simulink library "My_library"  (R2018a)
settings: Solver=VariableStepAuto  StartTime=0.0  StopTime=10.0  RelTol=1e-3  EnableMultiTasking=on
undefined symbols (not defined in the file or in its folder): Ax, Ay, Az, gn, Newton, Nx, Ny, Nz, Raphson, Rx, Ry, Rz, st
libraries: $bdroot x11, simulink x1
(part 1 of 2)
settings Model: Creator=Navya  LastModifiedBy=IGOSAT
settings DataIOCC: LimitDataPoints=on
settings OptimizationCC: LifeSpan=inf
settings DebuggingCC: AllowSymbolicDim=off  SFUnexpectedBacktrackingDiag=warning  SFNoUnconditionalDefaultTransitionDiag=warning  SFExecutionAtInitializationDiag=none
settings ModelReferenceCC: PropagateSignalLabelsOutOfModel=off
settings CodeAppCC: StateflowObjectComments=on
settings GRTTargetCC: TargetLangStandard=C89/C90 (ANSI)
settings ConfigComp: CovMetricSettings=dw  CovHtmlReporting=on  CovSaveCumulativeToWorkspaceVar=on  CovSaveSingleToWorkspaceVar=on  CovExternalEMLEnable=off

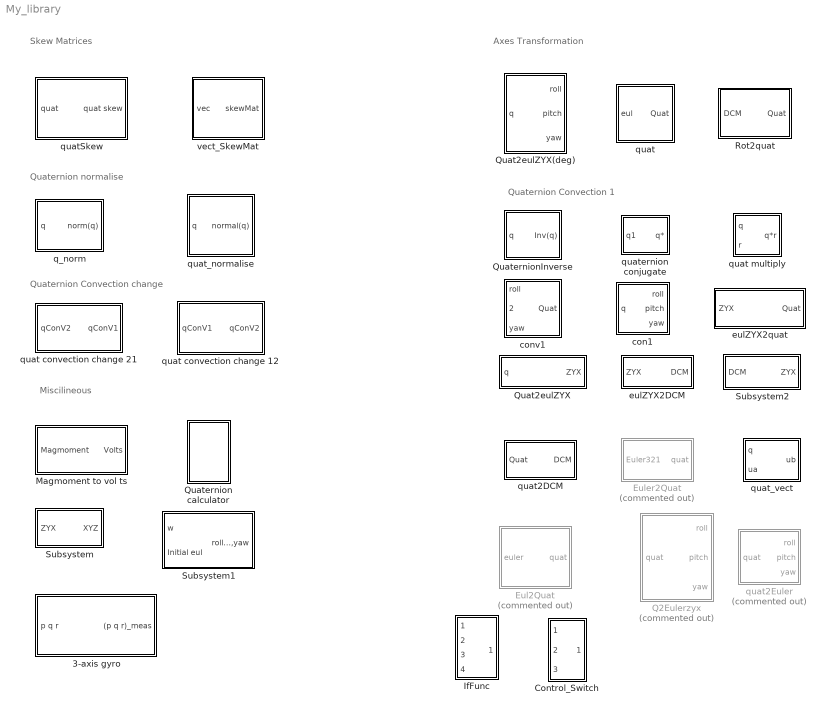
== system My_library ==
  note: Quaternion Convection 1
  note: Miscilineous
  note: Axes Transformation
  note: Quaternion Convection change
  note: Quaternion normalise
  note: Skew Matrices
  3-axis gyro : Subsystem  mask{dtype_g=off, w_g=190, z_g=0.707, g_sf_cc=[1 0 0; 0 1 0; 0 0 1], g_bias=1e-4*[1 1 1], g_sen=[0 0 0], g_Ts=0, Gs=0, g_rand=on, g_seeds=[23093 23094 23095], g_pow=gn, g_sat=[-inf  -inf  -inf  inf inf inf], ts=st}
      mask prompts: dtype_g "Second-order dynamics"; w_g "Natural frequency (rad/sec):"; z_g "Damping ratio:"; g_sf_cc "Scale factors and cross-coupling:"; g_bias "Measurement bias:"; g_sen "G-sensitive bias:"; g_Ts "Update rate (sec):"; Gs "Gyro sensitivity"; g_rand "Noise on:"; g_seeds "Noise seeds:"; g_pow "Noisepower:"; g_sat "Lower and upper output limits:"; ts "sampling time"
      mask init:
      | par = g_Ts;
      | block = gcb;
      | g_satl = g_sat(1:3);
      | g_sath = g_sat(4:6);
      | Ts=ts;
      mask DialogControl ParameterTabVar0 Prompt: Main
      mask DialogControl ParameterTabVar01 Prompt: Noise
      mask Display:
      | port_label('input',1,'w (rad/s)')
      | port_label('output',1,'w_meas (rad/s)')
  "Control_Switch " : Subsystem
  Eul2Quat : Subsystem  Commented=on
      mask help:
      | Converts euler(in deg) to Quaternion(of convection 2).
      | Input  : 3 x 1 [roll;pitch;yaw]
      | Output : 4 x 1
  Euler2Quat : Subsystem  Commented=on
      mask help: Convert euler321(in radians) to Quaternion of convection-2
  "IfFunc " : Subsystem
  Magmoment to vol ts : Subsystem
  Q2Eulerzyx : Subsystem  Commented=on
      mask help: Quaternion(convention 2) to euler(roll,pitch, yaw) in degress
  Quat2eulZYX : Subsystem
      mask help: Quaternion(Conv1) to euler ZYX(in rad)
  Quat2eulZYX(deg) : Subsystem
      mask help: Quaternion(convention 2) to euler(roll,pitch, yaw) in degress
  Quaternion calculator : Subsystem
      mask help: Calculates quaternion of convention-2 from euler angles
  QuaternionInverse : Subsystem
      mask help: Computes quaternion inverse for conv-1
  Rot2quat : Subsystem
      mask help: Rotation matrix to quaternion (conv-1)
  Subsystem : Subsystem
      mask help: Converts XYZ to ZYX format or viceversa
  Subsystem1 : Subsystem
      mask help: Computes euler angles (roll, pitch, yaw) from anguler rates(wx,wy,wz)
  Subsystem2 : Subsystem
      mask help: Converts DCM to euler ZYX
  con1 : Subsystem
      mask help: Quaternion(convention 1) to euler(roll,pitch, yaw) in degress
  conv1 : Subsystem
      mask help: roll pitch yaw(in rad) to quaternion conv-1 based on ZYX transformation
  eulZYX2DCM : Subsystem
      mask help: eulZYX(in rad) to DM
  eulZYX2quat : Subsystem
      mask help: euler ZYX(in rad) to Quaternion(Conv1).
  q_norm : Subsystem
      mask help:
      | Computes quaternion norm
      | norm(q) = q1^2+q2^2+q3^2+q4^2
  quat : Subsystem
      mask help:
      | Converts roll, pitch, yaw (in degress) to quaternion conv-2 based on eulZYX
      | Inputs: roll
      |         pitch
      |         yaw
      | Outputs:Quaternion [eps, eta]'
  quat convection change 12 : Subsystem
      mask help:
      | Changes the quaternion convection from 1 to 2
      | [q0;q1;q2;q3]->[q1;q2;q3;q4]
  quat convection change 21 : Subsystem
      mask help:
      | Changes the quaternion convection from 2 to 1
      | [q1;q2;q3;q4]->[q0;q1;q2;q3]
  quat multiply : Subsystem
      mask help:
      | quaternion multiplication (for conv-1)
      | qr = q*r
  quat2DCM : Subsystem
      mask help: Quaternion(conv - 1) to rotational matrix
  quat2Euler : Subsystem  Commented=on
      mask help: Converts quaternion(conv-2) to Euler Angles(in rad)
  quatSkew : Subsystem
      mask help: Compute quaternion skew matrix
  quat_normalise : Subsystem
      mask help:
      | Normalises the quaternion
      | normal(q)= q/√norm(q)
  quat_vect : Subsystem
      mask help:
      | If q is convention-1 and it tranforms vector from a to b.
      | ub = qba * ua
  quaternion conjugate : Subsystem
      mask help: Quaternion conjugate for convection-1
  vect_SkewMat : Subsystem
      mask help: Computes 3x3 skew matrix of a vector

== system My_library/3-axis gyro ==
  p q r : Inport  PortDimensions=3
  Measurement bias : Constant  Value=g_bias
  Product : Product  Multiplication=Matrix(*)  SaturateOnIntegerOverflow=on  OutDataTypeStr=Inherit: Same as first input
  Product1 : Product  SaturateOnIntegerOverflow=on  OutDataTypeStr=Inherit: Same as first input
  Random bias : simulink/Sources/Band-Limited White Noise  Cov=g_pow  Ts=Ts  seed=g_seeds(1:3)
  Saturation : Saturate  UpperLimit=g_sath  LowerLimit=g_satl
  "Scale factors & Cross-coupling errors " : Constant  Value=g_sf_cc
  Subsystem : Subsystem
  Sum1 : Sum  Inputs=|++  SaturateOnIntegerOverflow=on
  Sum4 : Sum  Inputs=+++  SaturateOnIntegerOverflow=on
  Zero-Order Hold : Gain  SaturateOnIntegerOverflow=on  OutDataTypeStr=Inherit: Same as input  ParamDataTypeStr=Inherit: Same as input
  Zero-Order Hold1 : Gain  SaturateOnIntegerOverflow=on  OutDataTypeStr=Inherit: Same as input  ParamDataTypeStr=Inherit: Same as input
  g-sensitive bias : Constant  Value=g_sen
  gyro sensitivity : Constant  Value=Gs
  (p q r)_meas : Outport
  wires:
  Sum4/1 -> Subsystem/1(p q r)
  "Scale factors & Cross-coupling errors "/1 -> Product/1
  p q r/1 -> Zero-Order Hold/1
  Subsystem/1("p q r ") -> Sum1/1
  Sum1/1 -> Saturation/1
  Zero-Order Hold/1 -> Product/2
  Saturation/1 -> (p q r)_meas/1
  g-sensitive bias/1 -> Product1/2
  Measurement bias/1 -> Sum4/2
  Product/1 -> Sum4/1
  Zero-Order Hold1/1 -> Product1/1
  Product1/1 -> Sum4/3
  gyro sensitivity/1 -> Zero-Order Hold1/1
  Random bias/1 -> Sum1/2

== system My_library/Control_Switch  ==
  In1 : Inport
  In2 : Inport  Port=2
  In3 : Inport  Port=3
  Control switch : Switch  Criteria=u2 ~= 0  Threshold=10000
  MATLAB Function2 : MATLAB Function  TreatAsAtomicUnit=on
  Out1 : Outport
  wires:
  In3/1 -> Control switch/3
  In1/1 -> Control switch/1
  In2/1 -> MATLAB Function2/1(x)
  Control switch/1 -> Out1/1
  MATLAB Function2/1(yes) -> Control switch/2

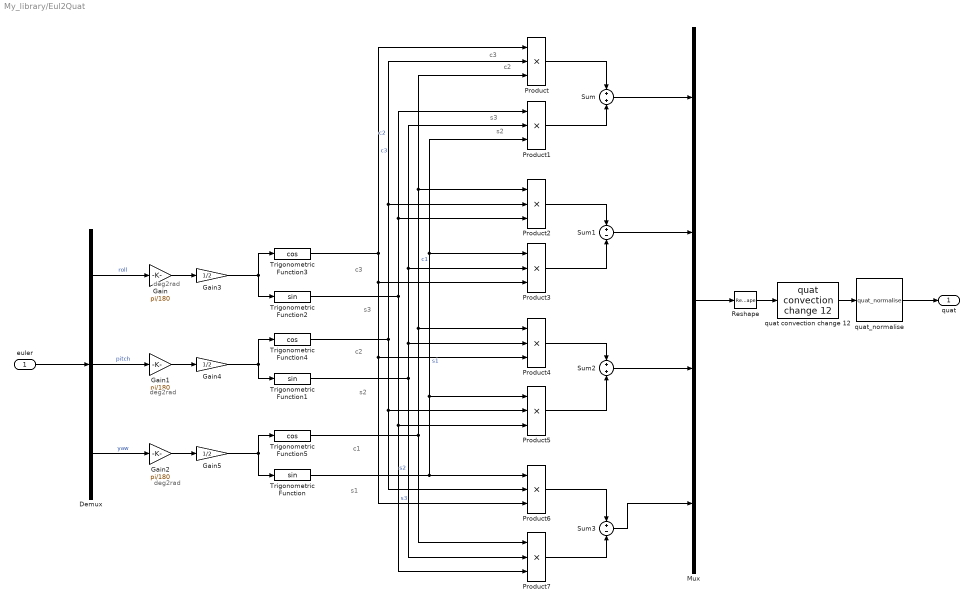
== system My_library/Eul2Quat ==
  note: deg2rad
  note: deg2rad
  note: deg2rad
  note: c2
  note: c3
  note: s2
  note: s3
  note: s1
  note: c1
  note: s2
  note: c2
  note: s3
  note: c3
  euler : Inport
  Demux : Demux  Outputs=3
  Gain : Gain  Gain=pi/180
  Gain1 : Gain  Gain=pi/180
  Gain2 : Gain  Gain=pi/180
  Gain3 : Gain  Gain=1/2
  Gain4 : Gain  Gain=1/2
  Gain5 : Gain  Gain=1/2
  Mux : Mux
  Product{,1..7} (8 alike) : Product  Inputs=3
  Reshape : Reshape
  Sum : Sum  Inputs=+|+
  Sum1 : Sum  Inputs=+|-
  Sum2 : Sum  Inputs=+|+
  Sum3 : Sum  Inputs=+|-
  Trigonometric Function : Trigonometry
  Trigonometric Function1 : Trigonometry
  Trigonometric Function2 : Trigonometry
  Trigonometric Function3 : Trigonometry  Operator=cos
  Trigonometric Function4 : Trigonometry  Operator=cos
  Trigonometric Function5 : Trigonometry  Operator=cos
  quat convection change 12 : $bdroot/quat convection change 12
  quat_normalise : $bdroot/quat_normalise
  quat : Outport
  wires:
  Gain1/1 -> Gain4/1
  Trigonometric Function2/1 -> Product2/3, Product1/1, Product7/3, Product5/3  "s3"
  Product2/1 -> Sum1/1
  Trigonometric Function3/1 -> Product/1, Product6/3, Product4/3, Product3/3  "c3"
  Sum/1 -> Mux/1
  Product3/1 -> Sum1/2
  Product1/1 -> Sum/2
  Product4/1 -> Sum2/1
  Trigonometric Function4/1 -> Product2/2, Product/2, Product6/2, Product5/2  "c2"
  Sum2/1 -> Mux/3
  Product7/1 -> Sum3/2
  Trigonometric Function1/1 -> Product4/2, Product1/2, Product3/2, Product7/2  "s2"
  Product/1 -> Sum/1
  Product6/1 -> Sum3/1
  Sum3/1 -> Mux/4
  Gain4/1 -> Trigonometric Function4/1, Trigonometric Function1/1
  Gain3/1 -> Trigonometric Function2/1, Trigonometric Function3/1
  Product5/1 -> Sum2/2
  Gain5/1 -> Trigonometric Function/1, Trigonometric Function5/1
  euler/1 -> Demux/1
  Mux/1 -> Reshape/1
  Trigonometric Function5/1 -> Product7/1, Product4/1, Product2/1, Product/3  "c1"
  Sum1/1 -> Mux/2
  Demux/1 -> Gain/1  "roll"
  Demux/3 -> Gain2/1  "yaw"
  Gain/1 -> Gain3/1
  Gain2/1 -> Gain5/1
  Trigonometric Function/1 -> Product3/1, Product1/3, Product5/1, Product6/1  "s1"
  Demux/2 -> Gain1/1  "pitch"
  Reshape/1 -> quat convection change 12/1
  quat convection change 12/1 -> quat_normalise/1
  quat_normalise/1 -> quat/1

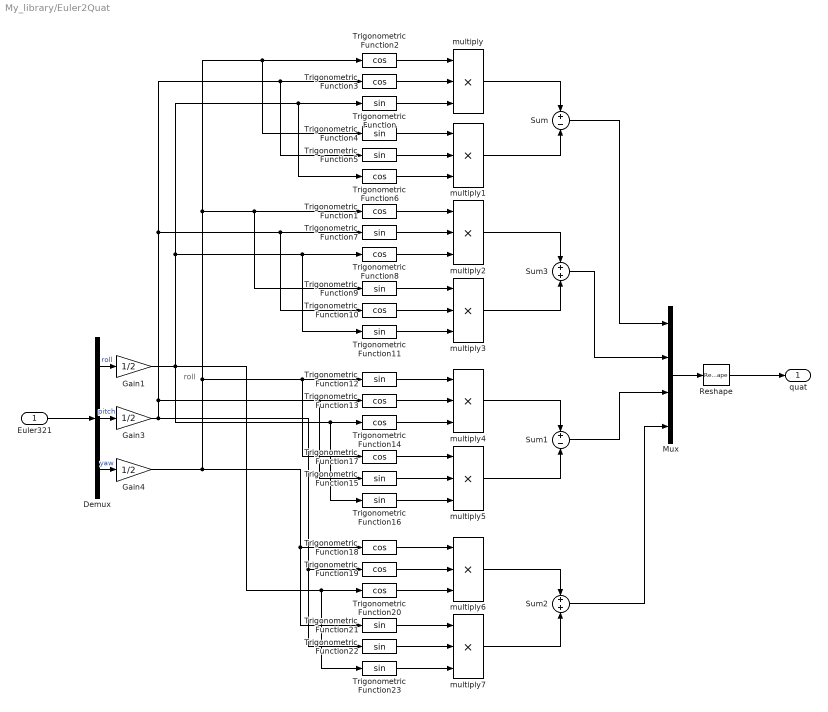
== system My_library/Euler2Quat ==
  note: roll
  Euler321 : Inport
  Demux : Demux  Outputs=3
  Gain1 : Gain  Gain=1/2
  Gain3 : Gain  Gain=1/2
  Gain4 : Gain  Gain=1/2
  Mux : Mux
  Reshape : Reshape
  Sum : Sum  Inputs=+-
  Sum1 : Sum  Inputs=+-
  Sum2 : Sum
  Sum3 : Sum
  Trigonometric Function{,4..5,7,9,11..12,15..16,21..23} (12 alike) : Trigonometry
  Trigonometric Function{1..3,6,8,10,13..14,17..20} (12 alike) : Trigonometry  Operator=cos
  multiply{,1..7} (8 alike) : Product  Inputs=***
  quat : Outport
  wires:
  Trigonometric Function1/1 -> multiply2/1
  Trigonometric Function9/1 -> multiply3/1
  Demux/2 -> Gain3/1  "pitch"
  multiply6/1 -> Sum2/1
  Euler321/1 -> Demux/1
  Trigonometric Function8/1 -> multiply2/3
  Demux/3 -> Gain4/1  "yaw"
  Trigonometric Function5/1 -> multiply1/2
  Trigonometric Function4/1 -> multiply1/1
  Trigonometric Function14/1 -> multiply4/3
  multiply1/1 -> Sum/2
  Trigonometric Function12/1 -> multiply4/1
  Trigonometric Function3/1 -> multiply/2
  Trigonometric Function13/1 -> multiply4/2
  Trigonometric Function6/1 -> multiply1/3
  Gain1/1 -> Trigonometric Function23/1, Trigonometric Function20/1, Trigonometric Function16/1, Trigonometric Function14/1, Trigonometric Function11/1, Trigonometric Function8/1, Trigonometric Function6/1, Trigonometric Function/1
  Gain3/1 -> Trigonometric Function22/1, Trigonometric Function19/1, Trigonometric Function15/1, Trigonometric Function13/1, Trigonometric Function10/1, Trigonometric Function7/1, Trigonometric Function5/1, Trigonometric Function3/1
  Gain4/1 -> Trigonometric Function21/1, Trigonometric Function18/1, Trigonometric Function17/1, Trigonometric Function12/1, Trigonometric Function4/1, Trigonometric Function2/1, Trigonometric Function9/1, Trigonometric Function1/1
  multiply7/1 -> Sum2/2
  Trigonometric Function23/1 -> multiply7/3
  Trigonometric Function2/1 -> multiply/1
  Mux/1 -> Reshape/1
  multiply3/1 -> Sum3/2
  Trigonometric Function16/1 -> multiply5/3
  Sum1/1 -> Mux/3
  Trigonometric Function22/1 -> multiply7/2
  multiply5/1 -> Sum1/2
  multiply/1 -> Sum/1
  Trigonometric Function15/1 -> multiply5/2
  Trigonometric Function17/1 -> multiply5/1
  Sum2/1 -> Mux/4
  Trigonometric Function10/1 -> multiply3/2
  Trigonometric Function21/1 -> multiply7/1
  Trigonometric Function/1 -> multiply/3
  multiply4/1 -> Sum1/1
  Reshape/1 -> quat/1
  Trigonometric Function18/1 -> multiply6/1
  Trigonometric Function20/1 -> multiply6/3
  Sum/1 -> Mux/1
  Trigonometric Function19/1 -> multiply6/2
  multiply2/1 -> Sum3/1
  Sum3/1 -> Mux/2
  Trigonometric Function7/1 -> multiply2/2
  Trigonometric Function11/1 -> multiply3/3
  Demux/1 -> Gain1/1  "roll"

== system My_library/IfFunc  ==
  In1 : Inport
  In2 : Inport  Port=2
  In3 : Inport  Port=3
  In4 : Inport  Port=4
  If : If  IfExpression=u1 == 2  ElseIfExpressions=u1 == 3, u1 ==1, u1 == 4
  If Action Subsystem : Subsystem  TreatAsAtomicUnit=on
  If Action Subsystem1 : Subsystem  TreatAsAtomicUnit=on
  If Action Subsystem2 : Subsystem  TreatAsAtomicUnit=on
  If Action Subsystem3 : Subsystem  TreatAsAtomicUnit=on
  If Action Subsystem4 : Subsystem  TreatAsAtomicUnit=on
  Merge : Merge  Inputs=5  InitialOutput=[0;0;0]
  Out1 : Outport
  wires:
  In2/1 -> If/1
  In3/1 -> If Action Subsystem3/1(In1), If Action Subsystem1/1(In1)
  If/1 -> If Action Subsystem/Action
  If/2 -> If Action Subsystem1/Action
  If/3 -> If Action Subsystem2/Action
  If Action Subsystem1/1(Out1) -> Merge/3
  If Action Subsystem2/1(Out1) -> Merge/5
  If Action Subsystem3/1(Out1) -> Merge/4
  If Action Subsystem4/1(Out1) -> Merge/2
  If Action Subsystem/1(Out1) -> Merge/1
  If/5 -> If Action Subsystem3/Action
  If/4 -> If Action Subsystem4/Action
  Merge/1 -> Out1/1
  In1/1 -> If Action Subsystem/1(In1)
  In4/1 -> If Action Subsystem2/1(In1)

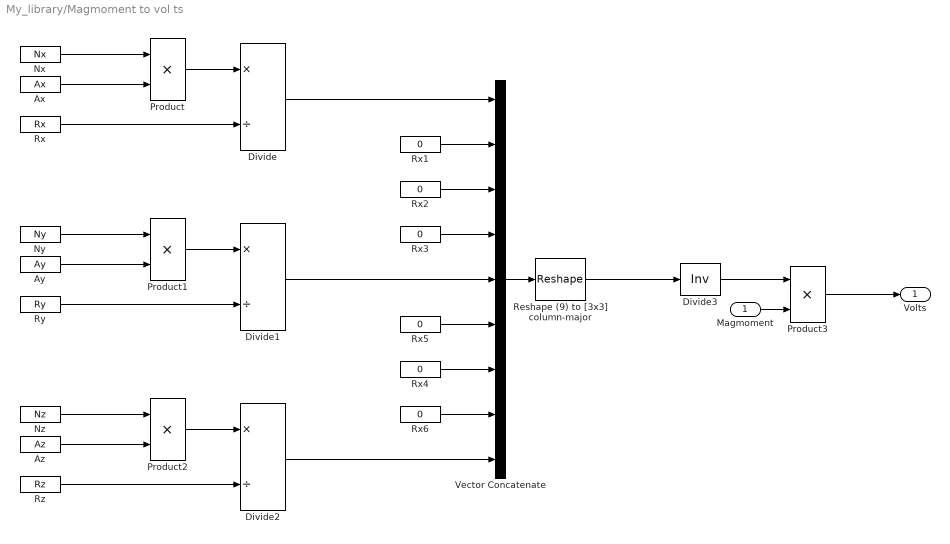
== system My_library/Magmoment to vol ts ==
  Magmoment : Inport
  Ax : Constant  Value=Ax
  Ay : Constant  Value=Ay
  Az : Constant  Value=Az
  Divide : Product  Inputs=*/
  Divide1 : Product  Inputs=*/
  Divide2 : Product  Inputs=*/
  Divide3 : Product  Inputs=/  Multiplication=Matrix(*)
  Nx : Constant  Value=Nx
  Ny : Constant  Value=Ny
  Nz : Constant  Value=Nz
  Product{,1..3} (4 alike) : Product
  Reshape (9) to [3x3] column-major : Reshape  OutputDimensionality=Customize  OutputDimensions=[3,3]
  Rx : Constant  Value=Rx
  Rx{1..6} (6 alike) : Constant  Value=0
  Ry : Constant  Value=Ry
  Rz : Constant  Value=Rz
  Vector Concatenate : Concatenate  NumInputs=9
  Volts : Outport
  wires:
  Vector Concatenate/1 -> Reshape (9) to [3x3] column-major/1
  Nx/1 -> Product/1
  Rz/1 -> Divide2/2
  Az/1 -> Product2/2
  Nz/1 -> Product2/1
  Product2/1 -> Divide2/1
  Ax/1 -> Product/2
  Product/1 -> Divide/1
  Product1/1 -> Divide1/1
  Ay/1 -> Product1/2
  Ny/1 -> Product1/1
  Ry/1 -> Divide1/2
  Rx6/1 -> Vector Concatenate/8
  Divide2/1 -> Vector Concatenate/9
  Rx2/1 -> Vector Concatenate/3
  Rx/1 -> Divide/2
  Divide1/1 -> Vector Concatenate/5
  Rx4/1 -> Vector Concatenate/7
  Rx3/1 -> Vector Concatenate/4
  Rx5/1 -> Vector Concatenate/6
  Rx1/1 -> Vector Concatenate/2
  Reshape (9) to [3x3] column-major/1 -> Divide3/1
  Divide/1 -> Vector Concatenate/1
  Divide3/1 -> Product3/1
  Magmoment/1 -> Product3/2
  Product3/1 -> Volts/1

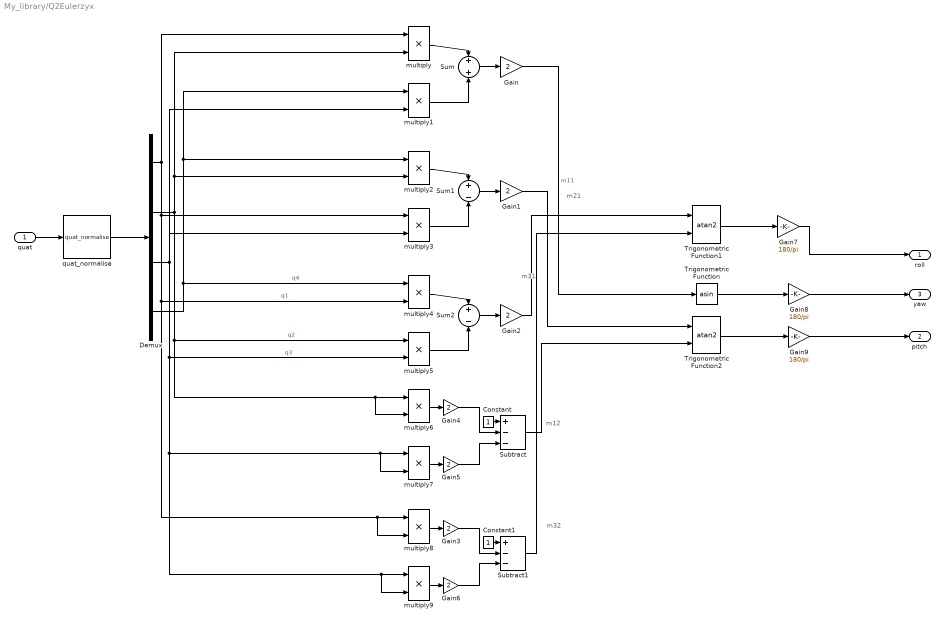
== system My_library/Q2Eulerzyx ==
  note: m21
  note: m12
  note: m32
  note: m31
  quat : Inport
  Constant : Constant
  Constant1 : Constant
  Demux : Demux
  Gain{,1..6} (7 alike) : Gain  Gain=2
  Gain7 : Gain  Gain=180/pi
  Gain8 : Gain  Gain=180/pi
  Gain9 : Gain  Gain=180/pi
  Subtract : Sum  Inputs=+--
  Subtract1 : Sum  Inputs=+--
  Sum : Sum  Inputs=+|+
  Sum1 : Sum  Inputs=+|-
  Sum2 : Sum  Inputs=+|-
  Trigonometric Function : Trigonometry  Operator=asin
  Trigonometric Function1 : Trigonometry  Operator=atan2
  Trigonometric Function2 : Trigonometry  Operator=atan2
  multiply{,1..9} (10 alike) : Product  Inputs=**
  quat_normalise : $bdroot/quat_normalise
  roll : Outport
  pitch : Outport  Port=2
  yaw : Outport  Port=3
  wires:
  Trigonometric Function/1 -> Gain8/1
  Trigonometric Function2/1 -> Gain9/1
  Gain/1 -> Trigonometric Function/1  "m11"
  Constant/1 -> Subtract/1
  Demux/2 -> multiply6/2, multiply6/1, multiply5/1, multiply2/2, multiply/2  "q2"
  multiply5/1 -> Sum2/2
  multiply1/1 -> Sum/2
  multiply8/1 -> Gain3/1
  Sum/1 -> Gain/1
  Trigonometric Function1/1 -> Gain7/1
  Subtract/1 -> Trigonometric Function2/2
  multiply/1 -> Sum/1
  multiply6/1 -> Gain4/1
  Gain2/1 -> Trigonometric Function1/1
  Gain4/1 -> Subtract/2
  Demux/1 -> multiply4/2, multiply8/2, multiply8/1, multiply3/1, multiply/1  "q1"
  Gain1/1 -> Trigonometric Function2/1
  Sum1/1 -> Gain1/1
  Subtract1/1 -> Trigonometric Function1/2
  multiply2/1 -> Sum1/1
  multiply4/1 -> Sum2/1
  Sum2/1 -> Gain2/1
  multiply3/1 -> Sum1/2
  Gain3/1 -> Subtract1/2
  Demux/3 -> multiply3/2, multiply7/2, multiply7/1, multiply9/2, multiply9/1, multiply5/2, multiply1/2  "q3"
  Gain7/1 -> roll/1
  Gain5/1 -> Subtract/3
  Demux/4 -> multiply4/1, multiply1/1, multiply2/1  "q4"
  Gain6/1 -> Subtract1/3
  Constant1/1 -> Subtract1/1
  Gain8/1 -> yaw/1
  quat/1 -> quat_normalise/1
  quat_normalise/1 -> Demux/1
  multiply7/1 -> Gain5/1
  multiply9/1 -> Gain6/1
  Gain9/1 -> pitch/1

== system My_library/Quat2eulZYX ==
  q : Inport
  Trigonometric Function1 : Trigonometry  Operator=atan2
  Trigonometric Function3 : Trigonometry  Operator=atan2
  Vector Concatenate : Concatenate  NumInputs=3
  fcn1 : Fcn  Expr=2*(u[2]*u[3] + u[1]*u[4])
  fcn2 : Fcn  Expr=u[1]*u[1] + u[2]*u[2] - u[3]*u[3] - u[4]*u[4]
  fcn3 : Fcn  Expr=-2*(u[2]*u[4] - u[1]*u[3])
  fcn4 : Fcn  Expr=2*(u[3]*u[4] + u[1]*u[2])
  fcn5 : Fcn  Expr=u[1]*u[1] - u[2]*u[2] - u[3]*u[3] + u[4]*u[4]
  quat_normalise : $bdroot/quat_normalise
  trigFcn : Trigonometry  Operator=asin
  ZYX : Outport
  wires:
  quat_normalise/1 -> fcn3/1, fcn4/1, fcn5/1, fcn2/1, fcn1/1
  Trigonometric Function3/1 -> Vector Concatenate/3  "r3"
  trigFcn/1 -> Vector Concatenate/2  "r2"
  Trigonometric Function1/1 -> Vector Concatenate/1  "r1"
  Vector Concatenate/1 -> ZYX/1
  q/1 -> quat_normalise/1
  fcn3/1 -> trigFcn/1
  fcn4/1 -> Trigonometric Function3/1
  fcn1/1 -> Trigonometric Function1/1
  fcn2/1 -> Trigonometric Function1/2
  fcn5/1 -> Trigonometric Function3/2

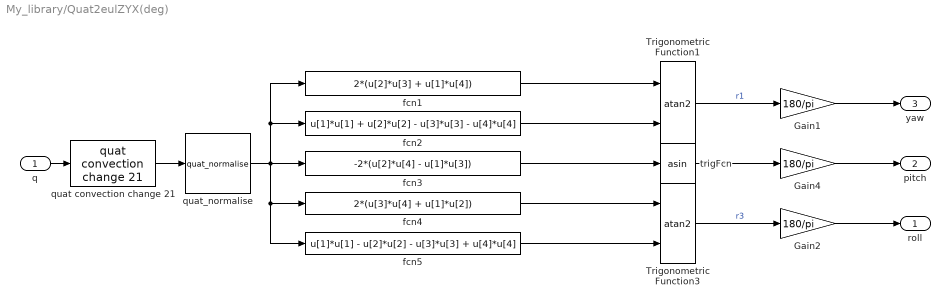
== system My_library/Quat2eulZYX(deg) ==
  q : Inport
  Gain1 : Gain  Gain=180/pi
  Gain2 : Gain  Gain=180/pi
  Gain4 : Gain  Gain=180/pi
  Trigonometric Function1 : Trigonometry  Operator=atan2
  Trigonometric Function3 : Trigonometry  Operator=atan2
  fcn1 : Fcn  Expr=2*(u[2]*u[3] + u[1]*u[4])
  fcn2 : Fcn  Expr=u[1]*u[1] + u[2]*u[2] - u[3]*u[3] - u[4]*u[4]
  fcn3 : Fcn  Expr=-2*(u[2]*u[4] - u[1]*u[3])
  fcn4 : Fcn  Expr=2*(u[3]*u[4] + u[1]*u[2])
  fcn5 : Fcn  Expr=u[1]*u[1] - u[2]*u[2] - u[3]*u[3] + u[4]*u[4]
  quat convection change 21 : $bdroot/quat convection change 21
  quat_normalise : $bdroot/quat_normalise
  trigFcn : Trigonometry  Operator=asin
  roll : Outport
  pitch : Outport  Port=2
  yaw : Outport  Port=3
  wires:
  Gain4/1 -> pitch/1
  trigFcn/1 -> Gain4/1
  Trigonometric Function1/1 -> Gain1/1  "r1"
  fcn2/1 -> Trigonometric Function1/2
  fcn4/1 -> Trigonometric Function3/1
  fcn5/1 -> Trigonometric Function3/2
  q/1 -> quat convection change 21/1
  fcn1/1 -> Trigonometric Function1/1
  fcn3/1 -> trigFcn/1
  quat_normalise/1 -> fcn3/1, fcn4/1, fcn5/1, fcn2/1, fcn1/1
  Trigonometric Function3/1 -> Gain2/1  "r3"
  Gain2/1 -> roll/1
  Gain1/1 -> yaw/1
  quat convection change 21/1 -> quat_normalise/1

== system My_library/Quaternion calculator ==
  note: q4
  note: q3
  note: q2
  note: q1
  note: Euler Angles (in deg)
  note: Quaternion
  " pitch" : Constant  Value=0
  " roll" : Constant  Value=0
  " yaw" : Constant  Value=0
  Demux : Demux
  Display{,1..3} (4 alike) : Display
  Eul2Quat1 : $bdroot/Eul2Quat
  Mux6 : Mux  Inputs=3
  wires:
  " roll"/1 -> Mux6/1
  Demux/3 -> Display2/1
  " yaw"/1 -> Mux6/3
  Demux/4 -> Display3/1
  Demux/2 -> Display1/1
  " pitch"/1 -> Mux6/2
  Mux6/1 -> Eul2Quat1/1
  Demux/1 -> Display/1
  Eul2Quat1/1 -> Demux/1

== system My_library/QuaternionInverse ==
  q : Inport
  Demux : Demux
  Divide{,1..3} (4 alike) : Product  Inputs=*/
  Mux : Mux
  q_norm : $bdroot/q_norm
  quaternion conjugate : Subsystem
      mask help: Quaternion conjugate for convection-1
  Inv(q) : Outport
  wires:
  Demux/2 -> Divide1/1
  Demux/3 -> Divide2/1
  Demux/4 -> Divide3/1
  Divide3/1 -> Mux/4
  Divide2/1 -> Mux/3
  Divide1/1 -> Mux/2
  Mux/1 -> Inv(q)/1
  Demux/1 -> Divide/1
  quaternion conjugate/1(q*) -> Demux/1
  q_norm/1 -> Divide/2, Divide1/2, Divide2/2, Divide3/2
  q/1 -> quaternion conjugate/1(q1), q_norm/1
  Divide/1 -> Mux/1

== system My_library/Rot2quat ==
  DCM : Inport  PortDimensions=[3,3]
  If : If
  Merge : Merge  InitialOutput=[1 0 0 0]
  Negative Trace : Subsystem  TreatAsAtomicUnit=on
  Positive Trace : Subsystem  TreatAsAtomicUnit=on
  "Reshape 3x3 -> 9" : Reshape  OutputDimensions=[9,1]
  Subsystem : Subsystem
  Quat : Outport  PortDimensions=4
  wires:
  Merge/1 -> Quat/1
  Subsystem/1(trace(DCM)) -> Positive Trace/1(trace(DCM)), If/1
  Negative Trace/1(qw qx qy qz) -> Merge/2
  If/2 -> Negative Trace/Action
  "Reshape 3x3 -> 9"/1 -> Positive Trace/2(DCM), Negative Trace/1(DCM), Subsystem/1(DCM)
  DCM/1 -> "Reshape 3x3 -> 9"/1
  Positive Trace/1(qw qx qy qz) -> Merge/1
  If/1 -> Positive Trace/Action

== system My_library/Subsystem ==
  ZYX : Inport
  Demux : Demux  Outputs=3
  Mux : Mux  Inputs=3
  XYZ : Outport
  wires:
  ZYX/1 -> Demux/1
  Demux/2 -> Mux/2
  Demux/1 -> Mux/3
  Mux/1 -> XYZ/1
  Demux/3 -> Mux/1

== system My_library/Subsystem1 ==
  w : Inport
  Initial eul : Inport  Port=2
  Demux : Demux  Outputs=3
  Integrator : Integrator  InitialConditionSource=external
  Subsystem1 : Subsystem
  Terminator : Terminator
  roll,pitch,yaw : Outport
  wires:
  Initial eul/1 -> Integrator/2
  w/1 -> Subsystem1/3(w)
  Subsystem1/1(rpydot) -> Integrator/1
  Demux/1 -> Subsystem1/1(phi)
  Demux/2 -> Subsystem1/2(theta)
  Demux/3 -> Terminator/1
  Integrator/1 -> roll,pitch,yaw/1, Demux/1

== system My_library/Subsystem2 ==
  DCM : Inport
  AxisRotDefault : Subsystem  TreatAsAtomicUnit=on
  AxisRotZeroR3 : Subsystem  TreatAsAtomicUnit=on
  Get DCM Values : Subsystem
  If : If  IfExpression=(u1>=1)|(u1<=-1)
  Merge : Merge
  Selector4 : Selector  InputPortWidth=7  IndexOptions=Index vector (dialog)  Indices=3  OutputSizes=1
  ZYX : Outport
  wires:
  AxisRotDefault/1(Out1) -> Merge/2
  Get DCM Values/1(Out1) -> AxisRotZeroR3/1(In1), AxisRotDefault/1(In1), Selector4/1
  Selector4/1 -> If/1  "r21"
  Merge/1 -> ZYX/1
  If/2 -> AxisRotDefault/Action
  If/1 -> AxisRotZeroR3/Action
  AxisRotZeroR3/1(Out1) -> Merge/1
  DCM/1 -> Get DCM Values/1(In1)

== system My_library/con1 ==
  q : Inport
  Gain1 : Gain  Gain=180/pi
  Gain2 : Gain  Gain=180/pi
  Gain4 : Gain  Gain=180/pi
  Trigonometric Function1 : Trigonometry  Operator=atan2
  Trigonometric Function3 : Trigonometry  Operator=atan2
  fcn1 : Fcn  Expr=2*(u[2]*u[3] + u[1]*u[4])
  fcn2 : Fcn  Expr=u[1]*u[1] + u[2]*u[2] - u[3]*u[3] - u[4]*u[4]
  fcn3 : Fcn  Expr=-2*(u[2]*u[4] - u[1]*u[3])
  fcn4 : Fcn  Expr=2*(u[3]*u[4] + u[1]*u[2])
  fcn5 : Fcn  Expr=u[1]*u[1] - u[2]*u[2] - u[3]*u[3] + u[4]*u[4]
  quat_normalise : $bdroot/quat_normalise
  trigFcn : Trigonometry  Operator=asin
  roll : Outport
  pitch : Outport  Port=2
  yaw : Outport  Port=3
  wires:
  Gain4/1 -> pitch/1
  trigFcn/1 -> Gain4/1
  Trigonometric Function1/1 -> Gain1/1  "r1"
  fcn2/1 -> Trigonometric Function1/2
  fcn4/1 -> Trigonometric Function3/1
  fcn5/1 -> Trigonometric Function3/2
  q/1 -> quat_normalise/1
  fcn1/1 -> Trigonometric Function1/1
  fcn3/1 -> trigFcn/1
  quat_normalise/1 -> fcn3/1, fcn4/1, fcn5/1, fcn2/1, fcn1/1
  Trigonometric Function3/1 -> Gain2/1  "r3"
  Gain2/1 -> roll/1
  Gain1/1 -> yaw/1

== system My_library/conv1 ==
  roll : Inport
  pitch : Inport  Port=2
  yaw : Inport  Port=3
  1/2 : Gain  Gain=0.5  SaturateOnIntegerOverflow=on  OutDataTypeStr=Inherit: Same as input  ParamDataTypeStr=Inherit: Same as input
  Mux1 : Mux  Inputs=2
  Mux2 : Mux
  Mux3 : Mux  Inputs=3
  q0 : Fcn  Expr=u(4)*u(5)*u(6) + u(1)*u(2)*u(3)
  q1 : Fcn  Expr=u(4)*u(5)*u(3) - u(1)*u(2)*u(6)
  q2 : Fcn  Expr=u(4)*u(2)*u(6) + u(1)*u(5)*u(3)
  q3 : Fcn  Expr=u(1)*u(5)*u(6) - u(4)*u(2)*u(3)
  sincos : Trigonometry  Operator=sincos
  Quat : Outport  InitialOutput=0
  wires:
  1/2/1 -> sincos/1
  Mux1/1 -> q0/1, q1/1, q2/1, q3/1
  q0/1 -> Mux2/1
  q1/1 -> Mux2/2
  q2/1 -> Mux2/3
  Mux2/1 -> Quat/1
  sincos/1 -> Mux1/1
  q3/1 -> Mux2/4
  sincos/2 -> Mux1/2
  yaw/1 -> Mux3/1
  roll/1 -> Mux3/3
  pitch/1 -> Mux3/2
  Mux3/1 -> 1/2/1

== system My_library/eulZYX2DCM ==
  ZYX : Inport  PortDimensions=3
  Fcn11 : Fcn  Expr=u(5)*u(4)
  Fcn12 : Fcn  Expr=u(5)*u(1)
  Fcn13 : Fcn  Expr=-u(2)
  Fcn21 : Fcn  Expr=u(3)*u(2)*u(4) - u(6)*u(1)
  Fcn22 : Fcn  Expr=u(3)*u(2)*u(1) + u(6)*u(4)
  Fcn23 : Fcn  Expr=u(3)*u(5)
  Fcn31 : Fcn  Expr=u(6)*u(2)*u(4) + u(3)*u(1)
  Fcn32 : Fcn  Expr=u(6)*u(2)*u(1) - u(3)*u(4)
  Fcn33 : Fcn  Expr=u(6)*u(5)
  Mux : Mux  Inputs=2
  Subsystem : Subsystem
  sincos : Trigonometry  Operator=sincos
  DCM : Outport  PortDimensions=[3,3]
  wires:
  ZYX/1 -> sincos/1
  Subsystem/1(Matrix) -> DCM/1
  sincos/1 -> Mux/1
  sincos/2 -> Mux/2
  Mux/1 -> Fcn11/1, Fcn12/1, Fcn13/1, Fcn21/1, Fcn32/1, Fcn33/1, Fcn31/1, Fcn23/1, Fcn22/1
  Fcn13/1 -> Subsystem/3(M13)
  Fcn31/1 -> Subsystem/7(M31)
  Fcn11/1 -> Subsystem/1(M11)
  Fcn21/1 -> Subsystem/4(M21)
  Fcn12/1 -> Subsystem/2(M12)
  Fcn22/1 -> Subsystem/5(M22)
  Fcn23/1 -> Subsystem/6(M23)
  Fcn32/1 -> Subsystem/8(M32)
  Fcn33/1 -> Subsystem/9(M33)

== system My_library/eulZYX2quat ==
  ZYX : Inport
  1/2 : Gain  Gain=0.5  SaturateOnIntegerOverflow=on  OutDataTypeStr=Inherit: Same as input  ParamDataTypeStr=Inherit: Same as input
  Mux1 : Mux  Inputs=2
  Mux2 : Mux
  q0 : Fcn  Expr=u(4)*u(5)*u(6) + u(1)*u(2)*u(3)
  q1 : Fcn  Expr=u(4)*u(5)*u(3) - u(1)*u(2)*u(6)
  q2 : Fcn  Expr=u(4)*u(2)*u(6) + u(1)*u(5)*u(3)
  q3 : Fcn  Expr=u(1)*u(5)*u(6) - u(4)*u(2)*u(3)
  sincos : Trigonometry  Operator=sincos
  Quat : Outport  InitialOutput=0
  wires:
  1/2/1 -> sincos/1
  sincos/1 -> Mux1/1
  Mux1/1 -> q0/1, q1/1, q2/1, q3/1
  q2/1 -> Mux2/3
  q3/1 -> Mux2/4
  Mux2/1 -> Quat/1
  ZYX/1 -> 1/2/1
  sincos/2 -> Mux1/2
  q0/1 -> Mux2/1
  q1/1 -> Mux2/2

== system My_library/q_norm ==
  q : Inport
  Demux : Demux
  Product{1..4} (4 alike) : Product
  Sum : Sum  Inputs=4
  norm(q) : Outport
  wires:
  Demux/1 -> Product1/1, Product1/2
  Demux/3 -> Product3/1, Product3/2
  Demux/2 -> Product2/1, Product2/2
  Product3/1 -> Sum/3
  Product4/1 -> Sum/4
  Product1/1 -> Sum/1
  Demux/4 -> Product4/1, Product4/2
  Product2/1 -> Sum/2
  q/1 -> Demux/1
  Sum/1 -> norm(q)/1

== system My_library/quat ==
  eul : Inport
  1/2 : Gain  Gain=0.5  SaturateOnIntegerOverflow=on  OutDataTypeStr=Inherit: Same as input  ParamDataTypeStr=Inherit: Same as input
  Demux : Demux  Outputs=3
  Gain : Gain  Gain=pi/180
  Mux1 : Mux  Inputs=2
  Mux2 : Mux
  Mux3 : Mux  Inputs=3
  q0 : Fcn  Expr=u(4)*u(5)*u(6) + u(1)*u(2)*u(3)
  q1 : Fcn  Expr=u(4)*u(5)*u(3) - u(1)*u(2)*u(6)
  q2 : Fcn  Expr=u(4)*u(2)*u(6) + u(1)*u(5)*u(3)
  q3 : Fcn  Expr=u(1)*u(5)*u(6) - u(4)*u(2)*u(3)
  sincos : Trigonometry  Operator=sincos
  Quat : Outport  InitialOutput=0
  wires:
  1/2/1 -> sincos/1
  Mux1/1 -> q0/1, q1/1, q2/1, q3/1
  q0/1 -> Mux2/1
  q1/1 -> Mux2/2
  q2/1 -> Mux2/3
  sincos/1 -> Mux1/1
  q3/1 -> Mux2/4
  sincos/2 -> Mux1/2
  Demux/3 -> Mux3/1
  Demux/1 -> Mux3/3
  Demux/2 -> Mux3/2
  Mux3/1 -> Gain/1
  Gain/1 -> 1/2/1
  Mux2/1 -> Quat/1
  eul/1 -> Demux/1

== system My_library/quat convection change 12 ==
  qConV1 : Inport
  Demux : Demux
  Mux : Mux
  qConV2 : Outport
  wires:
  Demux/4 -> Mux/3
  qConV1/1 -> Demux/1
  Mux/1 -> qConV2/1
  Demux/3 -> Mux/2
  Demux/2 -> Mux/1
  Demux/1 -> Mux/4

== system My_library/quat convection change 21 ==
  qConV2 : Inport
  Demux : Demux
  Mux : Mux
  qConV1 : Outport
  wires:
  Demux/1 -> Mux/2
  Demux/3 -> Mux/4
  Demux/2 -> Mux/3
  Demux/4 -> Mux/1
  qConV2/1 -> Demux/1
  Mux/1 -> qConV1/1

== system My_library/quat multiply ==
  q : Inport
  r : Inport  Port=2
  Mux : Mux
  q0 : Subsystem
  q1 : Subsystem
  q2 : Subsystem
  q3 : Subsystem
  q*r : Outport
  wires:
  Mux/1 -> q*r/1
  r/1 -> q0/2(r), q1/2(r), q3/2(r), q2/2(r)
  q3/1(q3) -> Mux/4
  q/1 -> q0/1(q), q1/1(q), q3/1(q), q2/1(q)
  q0/1(q0) -> Mux/1
  q1/1(q1) -> Mux/2
  q2/1(q2) -> Mux/3

== system My_library/quat2DCM ==
  Quat : Inport  PortDimensions=4
  Subsystem : Subsystem
  Subsystem1 : Subsystem
  Subsystem2 : Subsystem
  Subsystem3 : Subsystem
  Subsystem4 : Subsystem
  Subsystem5 : Subsystem
  Subsystem6 : Subsystem
  Subsystem7 : Subsystem
  Subsystem8 : Subsystem
  Subsystem9 : Subsystem
  DCM : Outport  PortDimensions=[3,3]  InitialOutput=0
  wires:
  Subsystem/1(Matrix) -> DCM/1
  Subsystem1/1(A11) -> Subsystem/1(M11)
  Subsystem4/1(A21) -> Subsystem/4(M21)
  Subsystem7/1(A31) -> Subsystem/7(M31)
  Subsystem8/1(A32) -> Subsystem/8(M32)
  Subsystem9/1(A33) -> Subsystem/9(M33)
  Quat/1 -> Subsystem1/1(normal(q)), Subsystem2/1(normal(q)), Subsystem3/1(normal(q)), Subsystem4/1(normal(q)), Subsystem5/1(normal(q)), Subsystem6/1(normal(q)), Subsystem7/1(normal(q)), Subsystem9/1(normal(q)), Subsystem8/1(normal(q))
  Subsystem5/1(A22) -> Subsystem/5(M22)
  Subsystem2/1(A12) -> Subsystem/2(M12)
  Subsystem3/1(A13) -> Subsystem/3(M13)
  Subsystem6/1(A23) -> Subsystem/6(M23)

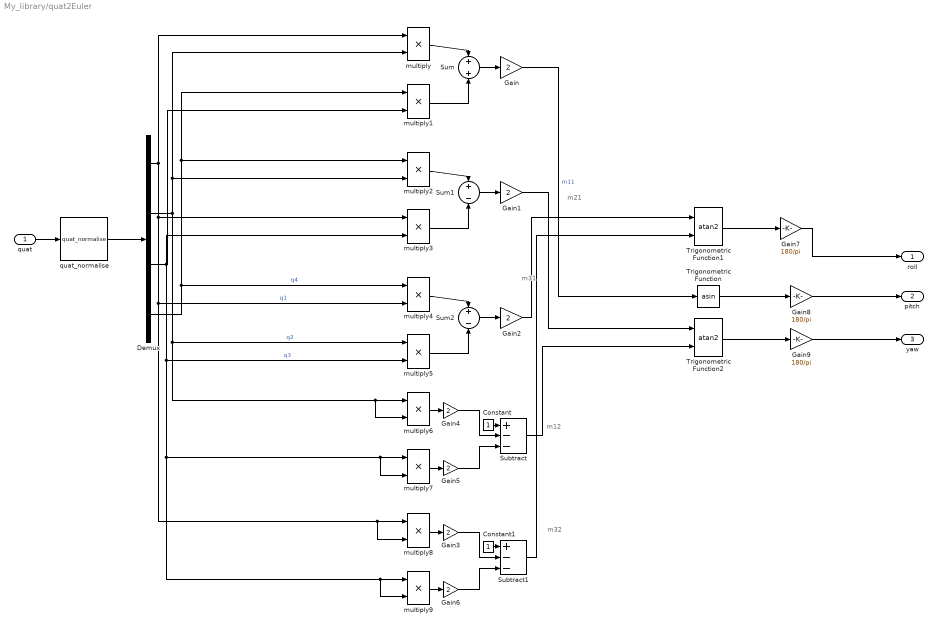
== system My_library/quat2Euler ==
  note: m21
  note: m12
  note: m32
  note: m31
  quat : Inport
  Constant : Constant
  Constant1 : Constant
  Demux : Demux
  Gain{,1..6} (7 alike) : Gain  Gain=2
  Gain7 : Gain  Gain=180/pi
  Gain8 : Gain  Gain=180/pi
  Gain9 : Gain  Gain=180/pi
  Subtract : Sum  Inputs=+--
  Subtract1 : Sum  Inputs=+--
  Sum : Sum  Inputs=+|+
  Sum1 : Sum  Inputs=+|-
  Sum2 : Sum  Inputs=+|-
  Trigonometric Function : Trigonometry  Operator=asin
  Trigonometric Function1 : Trigonometry  Operator=atan2
  Trigonometric Function2 : Trigonometry  Operator=atan2
  multiply{,1..9} (10 alike) : Product  Inputs=**
  quat_normalise : $bdroot/quat_normalise
  roll : Outport
  pitch : Outport  Port=2
  yaw : Outport  Port=3
  wires:
  multiply1/1 -> Sum/2
  Demux/2 -> multiply6/2, multiply6/1, multiply5/1, multiply2/2, multiply/2  "q2"
  Demux/1 -> multiply4/2, multiply8/2, multiply8/1, multiply3/1, multiply/1  "q1"
  Sum/1 -> Gain/1
  multiply/1 -> Sum/1
  Trigonometric Function2/1 -> Gain9/1
  Trigonometric Function/1 -> Gain8/1
  Gain1/1 -> Trigonometric Function2/1
  Trigonometric Function1/1 -> Gain7/1
  Sum2/1 -> Gain2/1
  Gain/1 -> Trigonometric Function/1  "m11"
  multiply2/1 -> Sum1/1
  multiply3/1 -> Sum1/2
  Sum1/1 -> Gain1/1
  multiply5/1 -> Sum2/2
  Gain2/1 -> Trigonometric Function1/1
  multiply4/1 -> Sum2/1
  multiply8/1 -> Gain3/1
  Subtract/1 -> Trigonometric Function2/2
  Gain4/1 -> Subtract/2
  Constant/1 -> Subtract/1
  multiply6/1 -> Gain4/1
  Subtract1/1 -> Trigonometric Function1/2
  multiply7/1 -> Gain5/1
  Gain3/1 -> Subtract1/2
  Gain5/1 -> Subtract/3
  multiply9/1 -> Gain6/1
  Gain6/1 -> Subtract1/3
  Constant1/1 -> Subtract1/1
  Demux/4 -> multiply4/1, multiply1/1, multiply2/1  "q4"
  Demux/3 -> multiply3/2, multiply7/2, multiply7/1, multiply9/2, multiply9/1, multiply5/2, multiply1/2  "q3"
  quat/1 -> quat_normalise/1
  quat_normalise/1 -> Demux/1
  Gain7/1 -> roll/1
  Gain9/1 -> yaw/1
  Gain8/1 -> pitch/1

== system My_library/quatSkew ==
  quat : Inport
  Demux1 : Demux
  Gain1 : Gain  Gain=-1
  Gain2 : Gain  Gain=-1
  Gain3 : Gain  Gain=-1
  Matrix Concatenate : Concatenate  NumInputs=4  Mode=Multidimensional array  ConcatenateDimension=2
  Mux{,1..3} (4 alike) : Mux
  Reshape{,1..3} (4 alike) : Reshape
  quat skew : Outport
  wires:
  Reshape/1 -> Matrix Concatenate/1
  Gain2/1 -> Mux1/4, Mux/3
  Mux2/1 -> Reshape2/1
  Mux/1 -> Reshape/1
  quat/1 -> Demux1/1
  Demux1/3 -> Mux3/3, Mux/2, Gain3/1
  Demux1/2 -> Mux3/2, Mux2/1, Gain2/1
  Matrix Concatenate/1 -> quat skew/1
  Gain1/1 -> Mux2/2, Mux/4
  Gain3/1 -> Mux2/4, Mux1/1
  Demux1/1 -> Mux3/1, Mux1/3, Gain1/1
  Mux1/1 -> Reshape1/1
  Reshape1/1 -> Matrix Concatenate/2
  Reshape2/1 -> Matrix Concatenate/3
  Reshape3/1 -> Matrix Concatenate/4
  Demux1/4 -> Mux3/4, Mux/1, Mux1/2, Mux2/3
  Mux3/1 -> Reshape3/1

== system My_library/quat_normalise ==
  q : Inport
  Demux : Demux
  Mux : Mux
  Product{1..4} (4 alike) : Product  Inputs=*/
  Reshape : Reshape
  "quat_modulus " : Subsystem
  normal(q) : Outport
  wires:
  Demux/4 -> Product4/1
  Demux/3 -> Product3/1
  Demux/2 -> Product2/1
  Demux/1 -> Product1/1
  q/1 -> "quat_modulus "/1(q), Demux/1
  "quat_modulus "/1(|q|) -> Product4/2, Product3/2, Product1/2, Product2/2
  Product1/1 -> Mux/1
  Product2/1 -> Mux/2
  Product3/1 -> Mux/3
  Product4/1 -> Mux/4
  Mux/1 -> Reshape/1
  Reshape/1 -> normal(q)/1

== system My_library/quat_vect ==
  q : Inport
  ua : Inport  Port=2
  Mux : Mux  Inputs=3
  V1 : Subsystem
  V2 : Subsystem
  V3 : Subsystem
  quat_normalise1 : $bdroot/quat_normalise
  ub : Outport
  wires:
  Mux/1 -> ub/1
  V3/1(V3) -> Mux/3
  V2/1(V2) -> Mux/2
  V1/1(V1) -> Mux/1
  ua/1 -> V1/2(vec1), V2/2(vec1), V3/2(vec1)
  q/1 -> quat_normalise1/1
  quat_normalise1/1 -> V1/1(q1), V2/1(q1), V3/1(q1)

== system My_library/quaternion conjugate ==
  q1 : Inport
  Demux1 : Demux
  Mux1 : Mux
  Unary Minus : UnaryMinus
  Unary Minus1 : UnaryMinus
  Unary Minus2 : UnaryMinus
  q* : Outport
  wires:
  Demux1/3 -> Unary Minus1/1
  Demux1/2 -> Unary Minus/1
  Unary Minus/1 -> Mux1/2
  Demux1/4 -> Unary Minus2/1
  Unary Minus1/1 -> Mux1/3
  Demux1/1 -> Mux1/1
  Mux1/1 -> q*/1
  q1/1 -> Demux1/1
  Unary Minus2/1 -> Mux1/4

== system My_library/vect_SkewMat ==
  vec : Inport
  Constant : Constant  Value=0
  Constant1 : Constant  Value=0
  Constant2 : Constant  Value=0
  Demux1 : Demux  Outputs=3
  Gain1 : Gain  Gain=-1
  Gain2 : Gain  Gain=-1
  Gain3 : Gain  Gain=-1
  Matrix Concatenate : Concatenate  NumInputs=3  Mode=Multidimensional array  ConcatenateDimension=2
  Mux : Mux  Inputs=3
  Mux1 : Mux  Inputs=3
  Mux2 : Mux  Inputs=3
  Reshape : Reshape
  Reshape1 : Reshape
  Reshape2 : Reshape
  skewMat : Outport
  wires:
  Reshape1/1 -> Matrix Concatenate/2
  Matrix Concatenate/1 -> skewMat/1
  Mux1/1 -> Reshape1/1
  Mux/1 -> Reshape/1
  Constant1/1 -> Mux1/2
  Demux1/1 -> Mux1/3, Gain1/1
  Gain2/1 -> Mux/3
  Constant/1 -> Mux/1
  vec/1 -> Demux1/1
  Reshape/1 -> Matrix Concatenate/1
  Reshape2/1 -> Matrix Concatenate/3
  Constant2/1 -> Mux2/3
  Gain1/1 -> Mux2/2
  Demux1/3 -> Mux/2, Gain3/1
  Mux2/1 -> Reshape2/1
  Demux1/2 -> Mux2/1, Gain2/1
  Gain3/1 -> Mux1/1

== system My_library/3-axis gyro/Subsystem ==
  p q r : Inport
  Constant : Constant  Value=dtype_g
  If : If  IfExpression=u1 == 1
  Merge : Merge  InitialOutput=[0; 0; 0]
  No dynamics : Subsystem  TreatAsAtomicUnit=on
  Second order dynamics : Subsystem  TreatAsAtomicUnit=on
  "p q r " : Outport
  wires:
  No dynamics/1(Out1) -> Merge/2
  Second order dynamics/1(Out1) -> Merge/1
  Merge/1 -> "p q r "/1
  Constant/1 -> If/1
  p q r/1 -> Second order dynamics/1(In1), No dynamics/1(In1)
  If/1 -> Second order dynamics/Action
  If/2 -> No dynamics/Action

== system My_library/IfFunc /If Action Subsystem ==
  In1 : Inport
  Action Port : ActionPort
  Out1 : Outport
  wires:
  In1/1 -> Out1/1

== system My_library/IfFunc /If Action Subsystem1 ==
  In1 : Inport
  Action Port : ActionPort
  Out1 : Outport
  wires:
  In1/1 -> Out1/1

== system My_library/IfFunc /If Action Subsystem2 ==
  In1 : Inport
  Action Port : ActionPort
  Out1 : Outport
  wires:
  In1/1 -> Out1/1

== system My_library/IfFunc /If Action Subsystem3 ==
  In1 : Inport
  Action Port : ActionPort
  Out1 : Outport
  wires:
  In1/1 -> Out1/1

== system My_library/IfFunc /If Action Subsystem4 ==
  Action Port : ActionPort
  Desired wx : Constant  Value=[0;0;0]
  Out1 : Outport
  wires:
  Desired wx/1 -> Out1/1

== system My_library/QuaternionInverse/quaternion conjugate ==
  q1 : Inport
  Demux1 : Demux
  Mux1 : Mux
  Unary Minus : UnaryMinus
  Unary Minus1 : UnaryMinus
  Unary Minus2 : UnaryMinus
  q* : Outport
  wires:
  Demux1/3 -> Unary Minus1/1
  Demux1/2 -> Unary Minus/1
  Unary Minus/1 -> Mux1/2
  Demux1/4 -> Unary Minus2/1
  Unary Minus1/1 -> Mux1/3
  Demux1/1 -> Mux1/1
  Mux1/1 -> q*/1
  q1/1 -> Demux1/1
  Unary Minus2/1 -> Mux1/4

== system My_library/Rot2quat/Negative Trace ==
  DCM : Inport
  Action Port : ActionPort
  Find Maximum Diagonal Value : If  NumInputs=3  IfExpression=((u2 > u1) & (u2 > u3))  ElseIfExpressions=u3 > u1
  "Maximum Value at DCM(1,1) " : Subsystem  TreatAsAtomicUnit=on
  Maximum Value at DCM(2,2) : Subsystem  TreatAsAtomicUnit=on
  "Maximum Value at DCM(3,3) " : Subsystem  TreatAsAtomicUnit=on
  Merge1 : Merge  Inputs=3
  diag(DCM) : Subsystem
  qw qx qy qz : Outport
  wires:
  diag(DCM)/3(u(9)) -> Find Maximum Diagonal Value/3
  diag(DCM)/2(u(5)) -> Find Maximum Diagonal Value/2
  diag(DCM)/1(u(1)) -> Find Maximum Diagonal Value/1
  DCM/1 -> diag(DCM)/1(DCM), Maximum Value at DCM(2,2)/1(DCM), "Maximum Value at DCM(1,1) "/1(DCM), "Maximum Value at DCM(3,3) "/1(DCM)
  Find Maximum Diagonal Value/3 -> "Maximum Value at DCM(1,1) "/Action
  Maximum Value at DCM(2,2)/1(qw qx qy qz) -> Merge1/1
  "Maximum Value at DCM(3,3) "/1(qw qx qy qz) -> Merge1/2
  "Maximum Value at DCM(1,1) "/1(qw qx qy qz) -> Merge1/3
  Merge1/1 -> qw qx qy qz/1
  Find Maximum Diagonal Value/1 -> Maximum Value at DCM(2,2)/Action
  Find Maximum Diagonal Value/2 -> "Maximum Value at DCM(3,3) "/Action

== system My_library/Rot2quat/Positive Trace ==
  trace(DCM) : Inport
  DCM : Inport  Port=2
  Action Port : ActionPort
  Constant1 : Constant  OutDataTypeStr=Inherit: Inherit via back propagation
  Gain : Gain  Gain=0.5  OutDataTypeStr=Inherit: Inherit via back propagation  SaturateOnIntegerOverflow=on  ParamDataTypeStr=Inherit: Same as input
  Gain1 : Gain  Gain=2  OutDataTypeStr=Inherit: Inherit via back propagation  SaturateOnIntegerOverflow=on  ParamDataTypeStr=Inherit: Same as input
  Mux : Mux  Inputs=2
  Mux1 : Mux  Inputs=3
  Product : Product  Inputs=*/  SaturateOnIntegerOverflow=on  InputSameDT=on  OutDataTypeStr=Inherit: Same as first input
  Sum1 : Sum  Inputs=++|  SaturateOnIntegerOverflow=on  InputSameDT=on  OutDataTypeStr=Inherit: Same as first input
  cos(phi)sin(theta)cos(psi) + sin(phi)sin(psi) +sin(theta) : Subsystem
  cos(theta)sin(phi) - (cos(phi)sin(theta)sin(psi) - sin(phi)cos(psi))1 : Subsystem
  cos(theta)sin(psi) - (sin(phi)sin(theta)cos(psi) - cos(phi)sin(psi))1 : Subsystem
  sqrt : Sqrt  AlgorithmType=Newton-Raphson  SaturateOnIntegerOverflow=on
  qw qx qy qz : Outport
  wires:
  trace(DCM)/1 -> Sum1/1
  cos(theta)sin(psi) - (sin(phi)sin(theta)cos(psi) - cos(phi)sin(psi))1/1(u(4)-u(2)) -> Mux1/3
  cos(theta)sin(phi) - (cos(phi)sin(theta)sin(psi) - sin(phi)cos(psi))1/1(u(8)-u(6)) -> Mux1/1
  sqrt/1 -> Gain/1, Gain1/1
  Mux/1 -> qw qx qy qz/1
  Sum1/1 -> sqrt/1
  Gain/1 -> Mux/1
  cos(phi)sin(theta)cos(psi) + sin(phi)sin(psi) +sin(theta)/1(u(3)-u(7)) -> Mux1/2
  Constant1/1 -> Sum1/2
  DCM/1 -> cos(phi)sin(theta)cos(psi) + sin(phi)sin(psi) +sin(theta)/1(DCM), cos(theta)sin(phi) - (cos(phi)sin(theta)sin(psi) - sin(phi)cos(psi))1/1(DCM), cos(theta)sin(psi) - (sin(phi)sin(theta)cos(psi) - cos(phi)sin(psi))1/1(DCM)
  Product/1 -> Mux/2
  Gain1/1 -> Product/2
  Mux1/1 -> Product/1

== system My_library/Rot2quat/Subsystem ==
  DCM : Inport
  Add : Sum  Inputs=+
  Selector : Selector  InputPortWidth=9  IndexOptions=Index vector (dialog)  Indices=[1 5 9]  OutputSizes=1
  trace(DCM) : Outport
  wires:
  Add/1 -> trace(DCM)/1
  DCM/1 -> Selector/1
  Selector/1 -> Add/1

== system My_library/Subsystem1/Subsystem1 ==
  phi : Inport
  theta : Inport  Port=2
  w : Inport  Port=3
  Product : Product  Multiplication=Matrix(*)
  Subsystem : Subsystem
  rpydot : Outport
  wires:
  Subsystem/1(J) -> Product/1
  w/1 -> Product/2
  Product/1 -> rpydot/1
  theta/1 -> Subsystem/2(theta)
  phi/1 -> Subsystem/1(phi)

== system My_library/Subsystem2/AxisRotDefault ==
  In1 : Inport
  Action Port : ActionPort
  Fcn1 : Fcn  Expr=atan2(u[1],u[2])
  Fcn2 : Fcn  Expr=asin(u[3])
  Fcn3 : Fcn  Expr=atan2(u[4],u[5])
  Vector Concatenate : Concatenate  NumInputs=3
  Out1 : Outport
  wires:
  Vector Concatenate/1 -> Out1/1
  Fcn3/1 -> Vector Concatenate/3  "r3"
  Fcn2/1 -> Vector Concatenate/2  "r2"
  Fcn1/1 -> Vector Concatenate/1  "r1"
  In1/1 -> Fcn2/1, Fcn1/1, Fcn3/1

== system My_library/Subsystem2/AxisRotZeroR3 ==
  In1 : Inport
  Action Port : ActionPort
  Fcn1 : Fcn  Expr=atan2(u[6],u[7])
  Fcn2 : Fcn  Expr=asin(u[3])
  Fcn3 : Fcn  Expr=0
  Vector Concatenate : Concatenate  NumInputs=3
  Out1 : Outport
  wires:
  In1/1 -> Fcn3/1, Fcn1/1, Fcn2/1
  Fcn1/1 -> Vector Concatenate/1  "r1"
  Fcn2/1 -> Vector Concatenate/2  "r2"
  Fcn3/1 -> Vector Concatenate/3  "r3"
  Vector Concatenate/1 -> Out1/1

== system My_library/Subsystem2/Get DCM Values ==
  In1 : Inport
  Gain1 : Gain  Gain=[1 1 -1]
  Gain2 : Gain  Gain=[1 1]
  Gain3 : Gain  Gain=[-1 1]
  Reshape : Reshape
  Reshape1 : Reshape
  Reshape2 : Reshape
  Selector1 : Selector  NumberOfDimensions=2  InputPortWidth=3  IndexOptions=Index vector (dialog),Index vector (dialog)  Indices=1,[2 1 3]  OutputSizes=1,1
  Selector2 : Selector  NumberOfDimensions=2  InputPortWidth=3  IndexOptions=Index vector (dialog),Index vector (dialog)  Indices=[2 3],3  OutputSizes=1,1
  Selector3 : Selector  NumberOfDimensions=2  InputPortWidth=3  IndexOptions=Index vector (dialog),Index vector (dialog)  Indices=2,[1 2]  OutputSizes=1,1
  Vector Concatenate : Concatenate  NumInputs=3
  Out1 : Outport
  wires:
  Selector1/1 -> Reshape/1
  Vector Concatenate/1 -> Out1/1
  Selector2/1 -> Reshape1/1
  Gain3/1 -> Vector Concatenate/3
  Gain1/1 -> Vector Concatenate/1
  In1/1 -> Selector3/1, Selector2/1, Selector1/1
  Reshape1/1 -> Gain2/1
  Reshape2/1 -> Gain3/1
  Reshape/1 -> Gain1/1
  Gain2/1 -> Vector Concatenate/2
  Selector3/1 -> Reshape2/1

== system My_library/eulZYX2DCM/Subsystem ==
  M11 : Inport  PortDimensions=1
  M12 : Inport  Port=2  PortDimensions=1
  M13 : Inport  Port=3  PortDimensions=1
  M21 : Inport  Port=4  PortDimensions=1
  M22 : Inport  Port=5  PortDimensions=1
  M23 : Inport  Port=6  PortDimensions=1
  M31 : Inport  Port=7  PortDimensions=1
  M32 : Inport  Port=8  PortDimensions=1
  M33 : Inport  Port=9  PortDimensions=1
  Reshape (9) to [3x3] column-major : Reshape  OutputDimensionality=Customize  OutputDimensions=[3,3]
  Vector Concatenate : Concatenate  NumInputs=9
  Matrix : Outport  PortDimensions=[3 3]
  wires:
  M32/1 -> Vector Concatenate/6
  M13/1 -> Vector Concatenate/7
  M33/1 -> Vector Concatenate/9
  M23/1 -> Vector Concatenate/8
  M11/1 -> Vector Concatenate/1
  Vector Concatenate/1 -> Reshape (9) to [3x3] column-major/1
  M21/1 -> Vector Concatenate/2
  M22/1 -> Vector Concatenate/5
  M31/1 -> Vector Concatenate/3
  M12/1 -> Vector Concatenate/4
  Reshape (9) to [3x3] column-major/1 -> Matrix/1

== system My_library/quat multiply/q0 ==
  q : Inport
  r : Inport  Port=2
  Demux : Demux
  Demux1 : Demux
  Product{,1..3} (4 alike) : Product  RndMeth=Zero
  Sum : Sum  Inputs=+---
  q0 : Outport
  wires:
  Demux1/4 -> Product3/2
  Demux1/3 -> Product2/2
  Demux/3 -> Product2/1
  Demux1/1 -> Product/2
  q/1 -> Demux/1
  Product2/1 -> Sum/3
  Product/1 -> Sum/1
  Demux1/2 -> Product1/2
  Product1/1 -> Sum/2
  Demux/4 -> Product3/1
  Product3/1 -> Sum/4
  Sum/1 -> q0/1
  r/1 -> Demux1/1
  Demux/2 -> Product1/1
  Demux/1 -> Product/1

== system My_library/quat multiply/q1 ==
  q : Inport
  r : Inport  Port=2
  Demux : Demux
  Demux1 : Demux
  Product{,1..3} (4 alike) : Product  RndMeth=Zero
  Sum : Sum  Inputs=+++-
  q1 : Outport
  wires:
  Demux1/4 -> Product2/2
  Product1/1 -> Sum/2
  Demux/1 -> Product/1
  Demux1/2 -> Product/2
  Demux1/1 -> Product1/2
  Demux/4 -> Product3/1
  Product2/1 -> Sum/3
  Product3/1 -> Sum/4
  Demux/3 -> Product2/1
  Demux1/3 -> Product3/2
  Sum/1 -> q1/1
  Product/1 -> Sum/1
  r/1 -> Demux1/1
  q/1 -> Demux/1
  Demux/2 -> Product1/1

== system My_library/quat multiply/q2 ==
  q : Inport
  r : Inport  Port=2
  Demux : Demux
  Demux1 : Demux
  Product{,1..3} (4 alike) : Product  RndMeth=Zero
  Sum : Sum  Inputs=+-++
  q2 : Outport
  wires:
  Demux1/1 -> Product2/2
  r/1 -> Demux1/1
  Demux1/2 -> Product3/2
  q/1 -> Demux/1
  Demux/3 -> Product2/1
  Product/1 -> Sum/1
  Demux/4 -> Product3/1
  Demux/1 -> Product/1
  Demux1/4 -> Product1/2
  Product2/1 -> Sum/3
  Demux1/3 -> Product/2
  Demux/2 -> Product1/1
  Sum/1 -> q2/1
  Product3/1 -> Sum/4
  Product1/1 -> Sum/2

== system My_library/quat multiply/q3 ==
  q : Inport
  r : Inport  Port=2
  Demux : Demux
  Demux1 : Demux
  Product{,1..3} (4 alike) : Product  RndMeth=Zero
  Sum : Sum  Inputs=++-+
  q3 : Outport
  wires:
  Product/1 -> Sum/1
  Demux/2 -> Product1/1
  Demux/1 -> Product/1
  q/1 -> Demux/1
  Demux/3 -> Product2/1
  Demux1/4 -> Product/2
  Sum/1 -> q3/1
  Demux/4 -> Product3/1
  Demux1/3 -> Product1/2
  r/1 -> Demux1/1
  Demux1/2 -> Product2/2
  Demux1/1 -> Product3/2
  Product1/1 -> Sum/2
  Product2/1 -> Sum/3
  Product3/1 -> Sum/4

== system My_library/quat2DCM/Subsystem ==
  M11 : Inport  PortDimensions=1
  M12 : Inport  Port=2  PortDimensions=1
  M13 : Inport  Port=3  PortDimensions=1
  M21 : Inport  Port=4  PortDimensions=1
  M22 : Inport  Port=5  PortDimensions=1
  M23 : Inport  Port=6  PortDimensions=1
  M31 : Inport  Port=7  PortDimensions=1
  M32 : Inport  Port=8  PortDimensions=1
  M33 : Inport  Port=9  PortDimensions=1
  Reshape (9) to [3x3] column-major : Reshape  OutputDimensionality=Customize  OutputDimensions=[3,3]
  Vector Concatenate : Concatenate  NumInputs=9
  Matrix : Outport  PortDimensions=[3 3]
  wires:
  M32/1 -> Vector Concatenate/6
  M13/1 -> Vector Concatenate/7
  M33/1 -> Vector Concatenate/9
  M23/1 -> Vector Concatenate/8
  M11/1 -> Vector Concatenate/1
  Vector Concatenate/1 -> Reshape (9) to [3x3] column-major/1
  M21/1 -> Vector Concatenate/2
  M22/1 -> Vector Concatenate/5
  M31/1 -> Vector Concatenate/3
  M12/1 -> Vector Concatenate/4
  Reshape (9) to [3x3] column-major/1 -> Matrix/1

== system My_library/quat2DCM/Subsystem1 ==
  normal(q) : Inport
  Demux : Demux
  Product{,1..3} (4 alike) : Product  RndMeth=Zero
  Sum : Sum  Inputs=++--
  A11 : Outport
  wires:
  Demux/2 -> Product2/1, Product2/2
  Product2/1 -> Sum/2
  Product3/1 -> Sum/1
  Product/1 -> Sum/4
  Product1/1 -> Sum/3
  Sum/1 -> A11/1
  Demux/3 -> Product1/1, Product1/2
  normal(q)/1 -> Demux/1
  Demux/1 -> Product3/1, Product3/2
  Demux/4 -> Product/1, Product/2

== system My_library/quat2DCM/Subsystem2 ==
  normal(q) : Inport
  Demux : Demux
  Gain : Gain  Gain=2
  Product2 : Product  RndMeth=Zero
  Product3 : Product  RndMeth=Zero
  Sum : Sum  Inputs=|++
  A12 : Outport
  wires:
  Sum/1 -> Gain/1
  normal(q)/1 -> Demux/1
  Gain/1 -> A12/1
  Product2/1 -> Sum/2
  Demux/1 -> Product3/2
  Product3/1 -> Sum/1
  Demux/4 -> Product3/1
  Demux/2 -> Product2/1
  Demux/3 -> Product2/2

== system My_library/quat2DCM/Subsystem3 ==
  normal(q) : Inport
  Demux : Demux
  Gain : Gain  Gain=2
  Product1 : Product  RndMeth=Zero
  Product2 : Product  RndMeth=Zero
  Sum : Sum  Inputs=|-+
  A13 : Outport
  wires:
  Demux/2 -> Product2/1
  Gain/1 -> A13/1
  Product2/1 -> Sum/2
  normal(q)/1 -> Demux/1
  Demux/3 -> Product1/2
  Product1/1 -> Sum/1
  Sum/1 -> Gain/1
  Demux/4 -> Product2/2
  Demux/1 -> Product1/1

== system My_library/quat2DCM/Subsystem4 ==
  normal(q) : Inport
  Demux : Demux
  Gain : Gain  Gain=2
  Product2 : Product  RndMeth=Zero
  Product3 : Product  RndMeth=Zero
  Sum : Sum  Inputs=|-+
  A21 : Outport
  wires:
  Product2/1 -> Sum/2
  normal(q)/1 -> Demux/1
  Product3/1 -> Sum/1
  Sum/1 -> Gain/1
  Demux/3 -> Product2/2
  Demux/4 -> Product3/1
  Demux/1 -> Product3/2
  Gain/1 -> A21/1
  Demux/2 -> Product2/1

== system My_library/quat2DCM/Subsystem5 ==
  normal(q) : Inport
  Demux : Demux
  Product{,1..3} (4 alike) : Product  RndMeth=Zero
  Sum : Sum  Inputs=+-+-
  A22 : Outport
  wires:
  Demux/2 -> Product2/2, Product2/1
  Sum/1 -> A22/1
  Product2/1 -> Sum/2
  Product1/1 -> Sum/3
  Demux/3 -> Product1/2, Product1/1
  Demux/4 -> Product/2, Product/1
  Demux/1 -> Product3/2, Product3/1
  Product3/1 -> Sum/1
  Product/1 -> Sum/4
  normal(q)/1 -> Demux/1

== system My_library/quat2DCM/Subsystem6 ==
  normal(q) : Inport
  Demux : Demux
  Gain : Gain  Gain=2
  Product1 : Product  RndMeth=Zero
  Product2 : Product  RndMeth=Zero
  Sum : Sum  Inputs=|++
  A23 : Outport
  wires:
  Gain/1 -> A23/1
  Product2/1 -> Sum/2
  Sum/1 -> Gain/1
  Demux/2 -> Product1/2
  Demux/4 -> Product2/2
  normal(q)/1 -> Demux/1
  Product1/1 -> Sum/1
  Demux/1 -> Product1/1
  Demux/3 -> Product2/1

== system My_library/quat2DCM/Subsystem7 ==
  normal(q) : Inport
  Demux : Demux
  Gain : Gain  Gain=2
  Product1 : Product  RndMeth=Zero
  Product2 : Product  RndMeth=Zero
  Sum : Sum  Inputs=|++
  A31 : Outport
  wires:
  Demux/3 -> Product1/2
  Demux/1 -> Product1/1
  Product1/1 -> Sum/1
  Sum/1 -> Gain/1
  normal(q)/1 -> Demux/1
  Product2/1 -> Sum/2
  Demux/2 -> Product2/1
  Demux/4 -> Product2/2
  Gain/1 -> A31/1

== system My_library/quat2DCM/Subsystem8 ==
  normal(q) : Inport
  Demux : Demux
  Gain : Gain  Gain=2
  Product1 : Product  RndMeth=Zero
  Product2 : Product  RndMeth=Zero
  Sum : Sum  Inputs=|-+
  A32 : Outport
  wires:
  Product1/1 -> Sum/1
  Sum/1 -> Gain/1
  Gain/1 -> A32/1
  Demux/3 -> Product2/1
  Demux/4 -> Product2/2
  Product2/1 -> Sum/2
  normal(q)/1 -> Demux/1
  Demux/2 -> Product1/2
  Demux/1 -> Product1/1

== system My_library/quat2DCM/Subsystem9 ==
  normal(q) : Inport
  Demux : Demux
  Product{,1..3} (4 alike) : Product  RndMeth=Zero
  Sum : Sum  Inputs=+--+
  A33 : Outport
  wires:
  Product3/1 -> Sum/1
  Product/1 -> Sum/4
  Demux/3 -> Product1/2, Product1/1
  Product2/1 -> Sum/2
  Product1/1 -> Sum/3
  Sum/1 -> A33/1
  Demux/1 -> Product3/2, Product3/1
  Demux/4 -> Product/2, Product/1
  normal(q)/1 -> Demux/1
  Demux/2 -> Product2/2, Product2/1

== system My_library/quat_normalise/quat_modulus  ==
  q : Inport
  q_norm : Subsystem
  sqrt : Sqrt  AlgorithmType=Newton-Raphson  SaturateOnIntegerOverflow=on
  |q| : Outport
  wires:
  q_norm/1(norm(q)) -> sqrt/1
  q/1 -> q_norm/1(q)
  sqrt/1 -> |q|/1
